simulink model "EuroNCAP_PedAEB"  (Simulink 10.0)
settings: Solver=VariableStepAuto  StartTime=0.0  StopTime=100  RelTol=1e-3
libraries: Solver_SF x1
settings Model: Creator=elowe  LastModifiedBy=elowe
settings DataIOCC: SaveFormat=Dataset  ReturnWorkspaceOutputs=on
settings OptimizationCC: LifeSpan=auto
settings DebuggingCC: UnderspecifiedInitializationDetection=Simplified  MergeDetectMultiDrivingBlocksExec=error  SFUnexpectedBacktrackingDiag=error  SFNoUnconditionalDefaultTransitionDiag=error  SFExecutionAtInitializationDiag=warning  ArithmeticOperatorsInVariantConditions=error
settings HardwareCC: ProdBitPerPointer=64  ProdBitPerSizeT=64  ProdBitPerPtrDiffT=64  ProdLargestAtomicFloat=Float  ProdIntDivRoundTo=Zero  ProdEndianess=LittleEndian  ProdWordSize=64  ProdHWDeviceType=Intel->x86-64 (Windows64)
settings ModelReferenceCC: PropagateSignalLabelsOutOfModel=on
settings SFSimCC: SimUseLocalCustomCode=on  CustomCodeUndefinedFunction=FilterOut
settings RTWCC: RTWUseLocalCustomCode=on
settings CodeAppCC: StateflowObjectComments=off
settings GRTTargetCC: TargetLangStandard=C99 (ISO)  CombineOutputUpdateFcns=on  GRTInterface=off
settings ConfigComp: CovMetricSettings=dwe  CovHtmlReporting=off  CovSaveCumulativeToWorkspaceVar=off  CovSaveSingleToWorkspaceVar=off

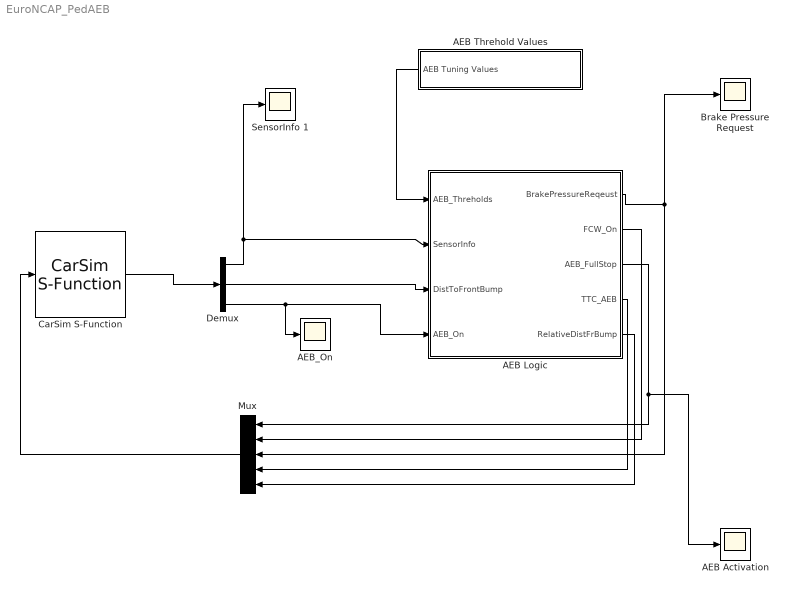
== system EuroNCAP_PedAEB ==
  AEB Activation : Scope
  AEB Logic : MATLAB Function  TreatAsAtomicUnit=on
  AEB Threhold Values : Subsystem
  AEB_On : Scope
  Brake Pressure Request : Scope
  CarSim S-Function : Solver_SF/CarSim S-Function  Priority=1  SIMFILE=simfile.sim  Run_RTs=off  vs_state_ind=Run  StopMode_ind=Vehicle Model
  Demux : Demux  Outputs=[4 1 1]
  Mux : Mux  Inputs=5
  SensorInfo 1 : Scope
  wires:
  AEB Threhold Values/1(AEB Tuning Values) -> AEB Logic/1(AEB_Threholds)
  AEB Logic/1(BrakePressureReqeust) -> Brake Pressure Request/1, Mux/3
  AEB Logic/2(FCW_On) -> Mux/2
  Demux/1 -> SensorInfo 1/1, AEB Logic/2(SensorInfo)
  Demux/2 -> AEB Logic/3(DistToFrontBump)
  AEB Logic/3(AEB_FullStop) -> AEB Activation/1, Mux/1
  Demux/3 -> AEB_On/1, AEB Logic/4(AEB_On)
  AEB Logic/4(TTC_AEB) -> Mux/4
  AEB Logic/5(RelativeDistFrBump) -> Mux/5
  Mux/1 -> CarSim S-Function/1
  CarSim S-Function/1 -> Demux/1

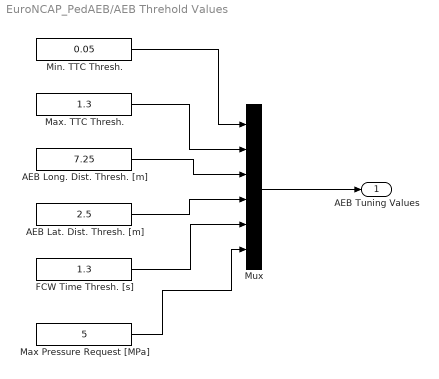
== system EuroNCAP_PedAEB/AEB Threhold Values ==
  AEB Lat. Dist. Thresh. [m] : Constant  Value=2.5
  AEB Long. Dist. Thresh. [m] : Constant  Value=7.25
  FCW Time Thresh. [s] : Constant  Value=1.3
  Max Pressure Request [MPa] : Constant  Value=5
  Max. TTC Thresh. : Constant  Value=1.3
  Min. TTC Thresh. : Constant  Value=0.05
  Mux : Mux  Inputs=6
  AEB Tuning Values : Outport
  wires:
  FCW Time Thresh. [s]/1 -> Mux/5
  Max. TTC Thresh./1 -> Mux/2
  AEB Lat. Dist. Thresh. [m]/1 -> Mux/4
  AEB Long. Dist. Thresh. [m]/1 -> Mux/3
  Mux/1 -> AEB Tuning Values/1
  Min. TTC Thresh./1 -> Mux/1
  Max Pressure Request [MPa]/1 -> Mux/6

== matlab function AEB Logic ==
  data: AEB_Threholds input double; BrakePressureReqeust output double; FCW_On output double; SensorInfo input double; DistToFrontBump input double; AEB_FullStop output double; AEB_On input double; TTC_AEB output double; RelativeDistFrBump output double
function [BrakePressureReqeust, FCW_On, AEB_FullStop,...
    TTC_AEB, RelativeDistFrBump] = AEB_SystemOutputs(AEB_Threholds,...
    SensorInfo, DistToFrontBump, AEB_On)

TTC_minTimeThresh = AEB_Threholds(1);
TTC_maxTimeThresh = AEB_Threholds(2);
AEB_longDistThresh = AEB_Threholds(3);
AEB_latDistThresh = AEB_Threholds(4);
FCW_timeThresh = AEB_Threholds(5);
MaxPressureReq = AEB_Threholds(6);

relDist = SensorInfo(1); % [m]: relative distance between the camera  
% and the detected object
relSpeed = SensorInfo(2); % [km/h]: relative speed between the camera 
% sensor and the object detected
relBearing = SensorInfo(3); % [deg] relative bearing between the camera 
% sensor and the detected object 
cameraObjDetect =  SensorInfo(4); % [-] boolean for when an object is 
% detected by the camera sensor

minDistThresh = 0.05; % [m]
distCamToFrBumper = DistToFrontBump; % [m] this is the known longitudinal 
% distance from the front bumper to the camera sensor 

FCW_On = 0;

longDistPedFtBump = 0; % [m]
latDistPedFtBump = 0; % [m]

relBearFrtBump = 0; % [rad]
relDistFrtBump = 0; % [m] relative distance from the front bumper along 
% the vehicle longitudinal axis, to the obstacle
RelativeDistFrBump = 0; % [m] output value, equivalent to relDistFrtBump

TTC_AEB = 0; % TTC calculation value [s]
AEB_TimeBool = 0; % boolean to know if AEB time threshold has been 
% satisfied for activation
AEB_DistBool = 0; % boolean to know if AEB distance threshold has been 
% satisfied for activation
AEB_FullStop = 0; % boolean for activating AEB, at maximum braking
FCW_On = 0; % boolean for activating FCW or not

if cameraObjDetect >= 1 
    longDistPedFtBump = relDist*cos(relBearing*(pi/180))-distCamToFrBumper;
    latDistPedFtBump =  relDist*sin(relBearing*(pi/180));
else
    longDistPedFtBump = 0;
    latDistPedFtBump =  0;
end

if abs(latDistPedFtBump) > minDistThresh
    relBearFrtBump = atan(latDistPedFtBump/longDistPedFtBump);
else
    relBearFrtBump = 0;
end

if abs(relBearFrtBump) > 0
    relDistFrtBump = latDistPedFtBump/sin(relBearFrtBump); 
    RelativeDistFrBump = relDistFrtBump;
else
    relDistFrtBump = 0;
    RelativeDistFrBump = relDistFrtBump;
end

% Time to collision from object to the ego vehicle's front bumper
if ( relSpeed < -TTC_minTimeThresh) && (cameraObjDetect >= 1)
    TTC_AEB =  abs(relDistFrtBump/(relSpeed/3.6));
else
    TTC_AEB =  0;
end
% TTC time threshold condition
if (TTC_AEB < TTC_maxTimeThresh) && (TTC_AEB > TTC_minTimeThresh)
    AEB_TimeBool = 1;
else
    AEB_TimeBool = 0;
end
% TTC distance threshold condition
if (longDistPedFtBump < AEB_longDistThresh) && ...
        (latDistPedFtBump < AEB_latDistThresh)
    AEB_DistBool = 1;
else
    AEB_DistBool = 0;
end

%*********************** AEB activation ***********************
if (cameraObjDetect >= 1)   % only apply AEB if the object is detected by 
                            % the camera sensor
    if (AEB_On == 1) && ((AEB_TimeBool == 1) || (AEB_DistBool == 1))
        AEB_FullStop = 1;
    else
        AEB_FullStop = 0; 
    end
end
BrakePressureReqeust = MaxPressureReq*AEB_FullStop;
%*********************** FCW activation ***********************
if (cameraObjDetect >= 1) && (relSpeed < 0) && (TTC_AEB < FCW_timeThresh)
    FCW_On = 1;
elseif AEB_FullStop == 1
    FCW_On = 1;
else
    FCW_On = 0;
end
